simulink model "state_feedback"  (R2023b)
settings: Solver=VariableStepAuto  StartTime=0.0  StopTime=20  RelTol=1e-3
values from neighbouring files (symbols this model uses):
  A = [0 1 0 0;0 0 1 0; 0 0 0 1;0 0 0 -5]    [statefeedback.m]
  B = [0;0;0;17]    [statefeedback.m]
  C = G/(P-G*P)    [statefeedback.m]
  K = place(A,B,P)    [statefeedback.m]
  Kr = 1 / Kdc    [statefeedback.m]
settings Model: Creator=DELL  LastModifiedBy=DELL

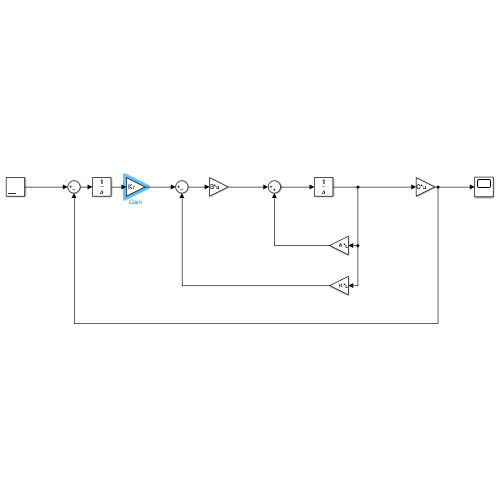
[thumbnail: Simulink's stored preview of the top-level diagram]
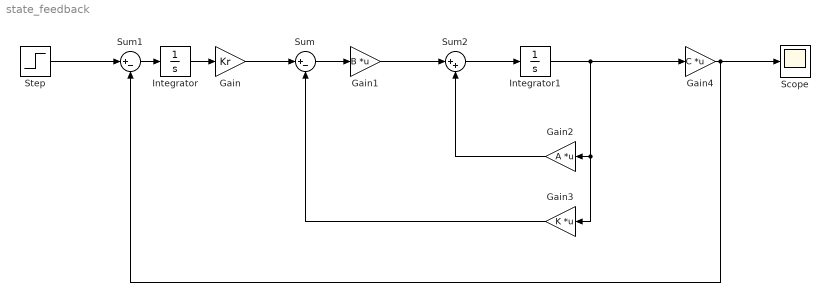
== system state_feedback ==
  Gain : Gain  Gain=Kr
  Gain1 : Gain  Gain=B  Multiplication=Matrix(K*u)
  Gain2 : Gain  Gain=A  Multiplication=Matrix(K*u)
  Gain3 : Gain  Gain=K  Multiplication=Matrix(K*u)
  Gain4 : Gain  Gain=C  Multiplication=Matrix(K*u)
  Integrator : Integrator
  Integrator1 : Integrator
  Scope : Scope
  Step : Step  Time=0  SampleTime=0
  Sum : Sum  Inputs=|+-
  Sum1 : Sum  Inputs=|+-
  Sum2 : Sum  Inputs=|++
  wires:
  Gain/1 -> Sum/1
  Step/1 -> Sum1/1
  Sum1/1 -> Integrator/1
  Integrator/1 -> Gain/1
  Sum/1 -> Gain1/1
  Gain1/1 -> Sum2/1
  Sum2/1 -> Integrator1/1
  Integrator1/1 -> Gain3/1, Gain2/1, Gain4/1
  Gain2/1 -> Sum2/2
  Gain3/1 -> Sum/2
  Gain4/1 -> Sum1/2, Scope/1
